simulink model "solver_simulink"  (R2016b)
settings: Solver=VariableStepAuto  StartTime=0.0  StopTime=10.0  RelTol=1e-3
values from neighbouring files (symbols this model uses):
  rINT = [0, site_elevation, 0]    [flightSimulation_simulink.m]    (also in initialconditions.m)
  T = 5e10    (= 50000000000)    [getAtmoConditions.m]    (also in getMotorData.m = interp1(t_thrust,thrust_curve,t_powered); initialconditions.m = [(0:t_step:motor.burntime)', T'])
  uINT = [0, 0, 0]    [flightSimulation_simulink.m]    (also in initialconditions.m)
settings Model: Creator=ME-123-10  LastModifiedBy=ME-123-10

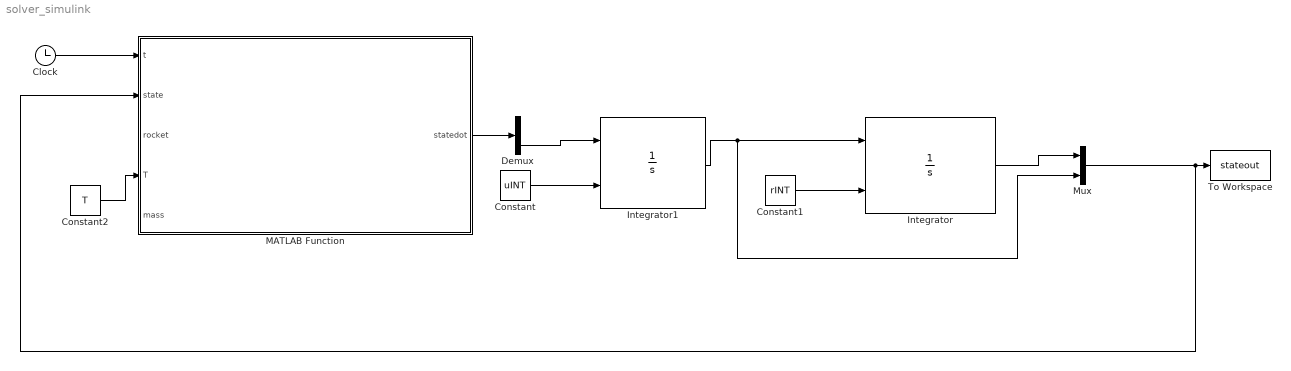
== system solver_simulink ==
  Clock : Clock
  Constant : Constant  Value=uINT
  Constant1 : Constant  Value=rINT
  Constant2 : Constant  Value=T
  Demux : Demux  Outputs=2
  Integrator : Integrator  InitialConditionSource=external
  Integrator1 : Integrator  InitialConditionSource=external
  MATLAB Function : MATLAB Function  TreatAsAtomicUnit=on
  Mux : Mux  Inputs=2
  To Workspace : ToWorkspace  VariableName=stateout  SampleTime=-1
  wires:
  Integrator1/1 -> Mux/2, Integrator/1
  Constant/1 -> Integrator1/2
  Constant1/1 -> Integrator/2
  Clock/1 -> MATLAB Function/1(t)
  MATLAB Function/1(statedot) -> Demux/1
  Demux/2 -> Integrator1/1
  Mux/1 -> To Workspace/1, MATLAB Function/2(state)
  Integrator/1 -> Mux/1
  Constant2/1 -> MATLAB Function/4(T)

== matlab function solver_simulink/MATLAB Function ==
  data: t input; statedot output; state input; rocket input; T input; mass input
function statedot = dot(t, state, rocket, T, mass)

% if rocket is at apogee, set theta = -180deg

statedot = zeros(6,1);  % initializes an empty vector
statedot(1:3) = state(4:6); % vx, vy, omega

% find force/acceleration; r = state(1:3); u = state(4:6)
[f_x, f_y, moment] = forces(rocket, t, state(1:3), state(4:6), T);

% lookup current mass and calculate moment of inertia
% current_mass = mass(t);

% find acceleration
a_x = f_x/current_mass; 
a_y = f_y/current_mass; 
alpha = moment/I;
statedot(4) = a_x; 
statedot(5) = a_y; 
statedot(6) = alpha;

end
